simulink model "Emission_Estimator_And_Consumption_Optimizer"  (R2016b)
settings: Solver=VariableStepAuto  StartTime=0.0  StopTime=10.0  RelTol=1e-3
libraries: gtlink2017 x1
settings Model: Creator=r03schne  LastModifiedBy=r03schne

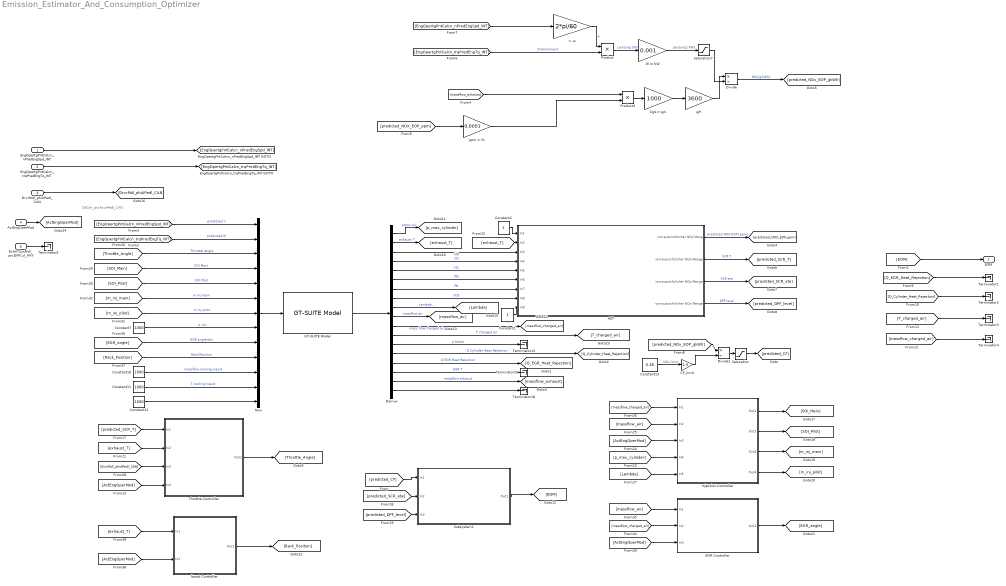
== system Emission_Estimator_And_Consumption_Optimizer ==
  note: DtCtrl_prcAccrPedl_CAN
  EngOpertgPntCalcn_nPredEngSpd_INT : Inport
  EngOpertgPntCalcn_trqPredEngTq_INT : Inport  Port=2
  DrvrMdl_phiAPedl_CAN : Inport  Port=3
  ActEngOperMod : Inport  Port=4
  ExhATSysMdl_prcDPFLvl_PHY : Inport  Port=5
  AET : Subsystem
      mask Display: image('C:\Users\r03schne\Pictures\RusspartikelFilter.jpg');
  "CF_limit " : Gain  Gain=1.5
  Constant1 : Constant
  Constant{7,10..12} (4 alike) : Constant  Value=1000
  Constant13 : Constant  Value=0.46
  Constant2 : Constant
  Demux : Demux  Outputs=18
  Divide : Product  Inputs=*/
  Divide1 : Product  Inputs=*/
  EGR Controller : Subsystem
      mask Display: image('C:\Users\r03schne\Pictures\drosselklappe_alt.png');
  GT-SUITE Model : gtlink2017/R2014b_and_higher /GT-SUITE Model  gti_fname='C:\Users\r03schne\Desktop\MAN_D26Dummymodell\D2676LF45_FRM_KF_BASIS_HARNESS-V2017.gtm'  gti_fname_warn=off  gti_dur=SIMULINK  gti_dt=0.001  gti_case=1  gti_ni=4  gti_no=18  gti_parnam='ign'  gti_parval='ign'  gti_runsimu=on  gti_coreno=1  gti_sui=console window  gti_monitors=on  gti_bits=default  gti_build=-1  gti_advanced=on  gti_halt=off  gti_initdlay=off  gti_cacomb=off  gti_ioreport=off  gti_feedthru=off  gti_add_image_to_block=Yes  gti_image_width=119  gti_image_height=139
      settings: AttributesFormatString=%<gti_fname>
  Injection Controller : Subsystem
      mask Display: image('C:\Users\r03schne\Pictures\injektor.png');
  Mux : Mux  Inputs=13
  Product : Product
  Product4 : Product
  Saturation : Saturate  UpperLimit=100  LowerLimit=0
  Saturation7 : Saturate  UpperLimit=4000  LowerLimit=1
  Subsystem1 : Subsystem
      mask Display: image('C:\Users\r03schne\Pictures\logic-1630657_960_720.png');
  Terminator{1..5,13,16,18} (8 alike) : Terminator
  Throttle Controller : Subsystem
      mask Display: image('C:\Users\r03schne\Pictures\drosselklappe_alt.png');
  W in KW : Gain  Gain=0.001
  boost Controller : Subsystem
      mask Display: image('C:\Users\r03schne\Pictures\GTX-Turbolader.jpg');
  g/h : Gain  Gain=3600
  kg/s in g/s : Gain  Gain=1000
  n -w : Gain  Gain=2*pi/60
  ppm in % : Gain  Gain=0.0001
  EOM : Outport  OutMin=0  OutMax=10  OutDataTypeStr=int8  PortDimensions="[1  1]"  SampleTime=0.01
  wires:
  GT-SUITE Model/1 -> Demux/1
  Demux/10 -> [massflow_air]  "massflow air"
  Demux/11 -> [massflow_charged_air]  "mass flow charged air"
  Mux/1 -> GT-SUITE Model/1
  Demux/12 -> [T_charged_air]  "T charged air"
  Demux/13 -> Terminator13/1  "p boost"
  Demux/14 -> [Q_Cylinder_Heat_Rejection]  "Q Cylinder Heat Rejection"
  Demux/15 -> [Q_EGR_Heat_Rejection]  "Q EGR Heat Rejection"
  Demux/16 -> Terminator16/1  "EGR T"
  Demux/17 -> [massflow_exhaust]  "massflow exhaust"
  Demux/18 -> Terminator18/1
  [Throttle_Angle] -> Mux/3  "Throttel Angle"
  [SOI_Main] -> Mux/4  "SOI Main"
  [SOI_Pilot] -> Mux/5  "SOI Pilot"
  [m_inj_main] -> Mux/6  "m inj main"
  [m_inj_pilot] -> Mux/7  "m inj pilot"
  Constant7/1 -> Mux/8  "p rail"
  [EGR_angle] -> Mux/9  "EGR angle/dm"
  [Rack_Position] -> Mux/10  "Rack-Position"
  Constant10/1 -> Mux/11  "massflow cooling_liquid"
  Constant11/1 -> Mux/12  "T cooling liquid"
  Constant12/1 -> Mux/13
  Demux/1 -> [p_max_cylinder]  "pmax cyl"
  Demux/2 -> [exhaust_T]  "exhaust T"
  Demux/3 -> AET/3(In3)  "NO"
  Demux/4 -> AET/4(In4)  "CO"
  Demux/5 -> AET/5(In5)  "HC"
  Demux/6 -> AET/6(In6)  "PM"
  Demux/7 -> AET/7(In7)  "PN"
  Demux/8 -> AET/8(In8)  "CO2"
  Demux/9 -> [Lambda]  "Lambda"
  Constant13/1 -> "CF_limit "/1  "NOx limit"
  AET/1(vorraussichtlicher NOx Menge) -> [predicted_NOX_EOP_ppm]  "predicted NOX EOP [ppm]"
  n -w/1 -> Product/1  "w"
  Product/1 -> W in KW/1  "Leistung [W]"
  [EngOpertgPntCalcn_trqPredEngTq_INT] -> Product/2  "Drehmoment"
  W in KW/1 -> Saturation7/1  "Leistung [KW]"
  ppm in %/1 -> Product4/2
  Product4/1 -> kg/s in g/s/1
  kg/s in g/s/1 -> g/h/1
  g/h/1 -> Divide/1
  Divide/1 -> [predicted_NOx_EOP_gkWh]  "NOx[g/kWh]"
  [massflow_exhaust] -> Product4/1
  Saturation7/1 -> Divide/2
  [EngOpertgPntCalcn_nPredEngSpd_INT] -> n -w/1
  [predicted_NOX_EOP_ppm] -> ppm in %/1
  [predicted_NOx_EOP_gkWh] -> Divide1/1
  "CF_limit "/1 -> Divide1/2
  Divide1/1 -> Saturation/1
  Saturation/1 -> [predicted_CF]
  AET/2(vorraussichtlicher NOx Menge1) -> [predicted_SCR_T]  "SCR T"
  AET/3(vorraussichtlicher NOx Menge2) -> [predicted_SCR_eta]  "SCR eta"
  AET/4(vorraussichtlicher NOx Menge3) -> [predicted_DPF_level]  "DPF level"
  [predicted_SCR_T] -> Throttle Controller/1(In1)
  [exhaust_T] -> Throttle Controller/2(In2)
  Throttle Controller/1(Out1) -> [Throttle_Angle]
  [exhaust_T] -> AET/2(In2)
  DrvrMdl_phiAPedl_CAN/1 -> [DrvrMdl_phiAPedl_CAN]
  [DrvrMdl_phiAPedl_CAN] -> Throttle Controller/3(In3)
  [massflow_charged_air] -> Injection Controller/1(In1)
  [massflow_air] -> Injection Controller/2(In2)
  [ActEngOperMod] -> Injection Controller/3(In3)
  [p_max_cylinder] -> Injection Controller/4(In4)
  [Lambda] -> Injection Controller/5(In5)
  Injection Controller/1(Out1) -> [SOI_Main]
  Injection Controller/2(Out2) -> [SOI_Pilot]
  Injection Controller/3(Out3) -> [m_inj_main]
  Injection Controller/4(Out4) -> [m_inj_pilot]
  [massflow_air] -> EGR Controller/1(In1)
  [massflow_charged_air] -> EGR Controller/2(In2)
  [ActEngOperMod] -> EGR Controller/3(In3)
  EGR Controller/1(Out1) -> [EGR_angle]
  [exhaust_T] -> boost Controller/1(In1)
  [ActEngOperMod] -> boost Controller/2(In2)
  boost Controller/1(Out1) -> [Rack_Position]
  Subsystem1/1(Out1) -> [EOM]
  [predicted_CF] -> Subsystem1/1(In1)
  [EOM] -> EOM/1
  EngOpertgPntCalcn_nPredEngSpd_INT/1 -> [EngOpertgPntCalcn_nPredEngSpd_INT]
  EngOpertgPntCalcn_trqPredEngTq_INT/1 -> [EngOpertgPntCalcn_trqPredEngTq_INT]
  [EngOpertgPntCalcn_nPredEngSpd_INT] -> Mux/1  "predicted n"
  [EngOpertgPntCalcn_trqPredEngTq_INT] -> Mux/2  "predicted M"
  Constant2/1 -> AET/1(In1)
  [massflow_charged_air] -> Terminator4/1
  Constant1/1 -> AET/9(In9)
  [Q_Cylinder_Heat_Rejection] -> Terminator2/1
  [Q_EGR_Heat_Rejection] -> Terminator1/1
  [T_charged_air] -> Terminator3/1
  [predicted_SCR_eta] -> Subsystem1/2(In2)
  [predicted_DPF_level] -> Subsystem1/3(In3)
  ActEngOperMod/1 -> [ActEngOperMod]
  [ActEngOperMod] -> Throttle Controller/4(In4)
  ExhATSysMdl_prcDPFLvl_PHY/1 -> Terminator5/1

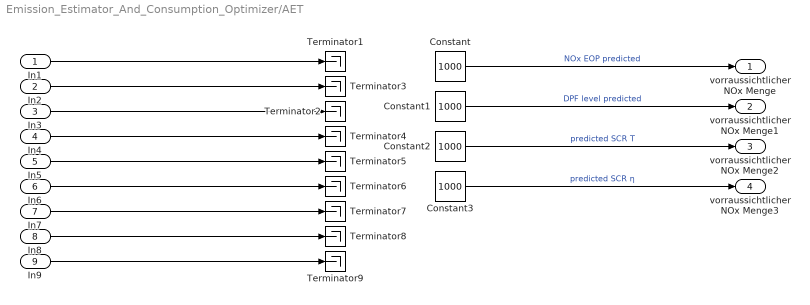
== system Emission_Estimator_And_Consumption_Optimizer/AET ==
  In1 : Inport
  In2 : Inport  Port=2
  In3 : Inport  Port=3
  In4 : Inport  Port=4
  In5 : Inport  Port=5
  In6 : Inport  Port=6
  In7 : Inport  Port=7
  In8 : Inport  Port=8
  In9 : Inport  Port=9
  Constant{,1..3} (4 alike) : Constant  Value=1000
  Terminator{1..9} (9 alike) : Terminator
  vorraussichtlicher NOx Menge : Outport
  vorraussichtlicher NOx Menge1 : Outport  Port=2
  vorraussichtlicher NOx Menge2 : Outport  Port=3
  vorraussichtlicher NOx Menge3 : Outport  Port=4
  wires:
  In3/1 -> Terminator2/1
  In2/1 -> Terminator3/1
  In4/1 -> Terminator4/1
  In5/1 -> Terminator5/1
  In6/1 -> Terminator6/1
  In7/1 -> Terminator7/1
  In8/1 -> Terminator8/1
  In9/1 -> Terminator9/1
  In1/1 -> Terminator1/1
  Constant1/1 -> vorraussichtlicher NOx Menge1/1  "DPF level predicted"
  Constant/1 -> vorraussichtlicher NOx Menge/1  "NOx EOP predicted"
  Constant2/1 -> vorraussichtlicher NOx Menge2/1  "predicted SCR T"
  Constant3/1 -> vorraussichtlicher NOx Menge3/1  "predicted SCR η"

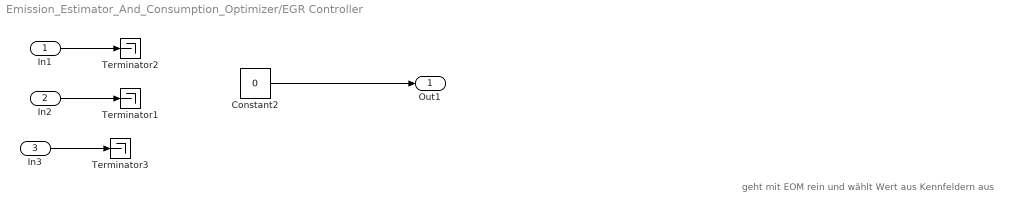
== system Emission_Estimator_And_Consumption_Optimizer/EGR Controller ==
  note: geht mit EOM rein und wählt Wert aus Kennfeldern aus
  In1 : Inport
  In2 : Inport  Port=2
  In3 : Inport  Port=3
  Constant2 : Constant  Value=0
  Terminator1 : Terminator
  Terminator2 : Terminator
  Terminator3 : Terminator
  Out1 : Outport
  wires:
  Constant2/1 -> Out1/1
  In3/1 -> Terminator3/1
  In2/1 -> Terminator1/1
  In1/1 -> Terminator2/1

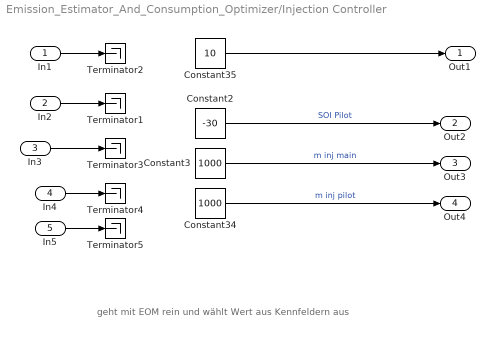
== system Emission_Estimator_And_Consumption_Optimizer/Injection Controller ==
  note: geht mit EOM rein und wählt Wert aus Kennfeldern aus
  In1 : Inport
  In2 : Inport  Port=2
  In3 : Inport  Port=3
  In4 : Inport  Port=4
  In5 : Inport  Port=5
  Constant2 : Constant  Value=-30
  Constant3 : Constant  Value=1000
  Constant34 : Constant  Value=1000
  Constant35 : Constant  Value=10
  Terminator{1..5} (5 alike) : Terminator
  Out1 : Outport
  Out2 : Outport  Port=2
  Out3 : Outport  Port=3
  Out4 : Outport  Port=4
  wires:
  Constant35/1 -> Out1/1
  Constant3/1 -> Out3/1  "m inj main"
  Constant34/1 -> Out4/1  "m inj pilot"
  Constant2/1 -> Out2/1  "SOI Pilot"
  In5/1 -> Terminator5/1
  In3/1 -> Terminator3/1
  In4/1 -> Terminator4/1
  In1/1 -> Terminator2/1
  In2/1 -> Terminator1/1

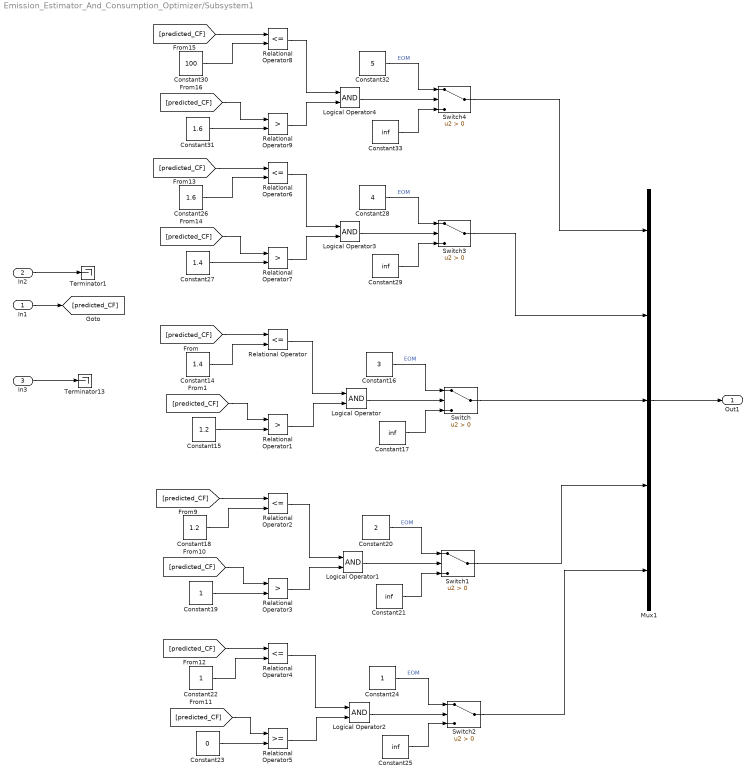
== system Emission_Estimator_And_Consumption_Optimizer/Subsystem1 ==
  In1 : Inport
  In2 : Inport  Port=2
  In3 : Inport  Port=3
  Constant14 : Constant  Value=1.4
  Constant15 : Constant  Value=1.2
  Constant16 : Constant  Value=3
  Constant{17,21,25,29,33} (5 alike) : Constant  Value=inf
  Constant18 : Constant  Value=1.2
  Constant19 : Constant
  Constant20 : Constant  Value=2
  Constant22 : Constant
  Constant23 : Constant  Value=0
  Constant24 : Constant
  Constant26 : Constant  Value=1.6
  Constant27 : Constant  Value=1.4
  Constant28 : Constant  Value=4
  Constant30 : Constant  Value=100
  Constant31 : Constant  Value=1.6
  Constant32 : Constant  Value=5
  Logical Operator{,1..4} (5 alike) : Logic  AllPortsSameDT=off  OutDataTypeStr=boolean
  Mux1 : Mux  Inputs=5
  Relational Operator{,2,4,6,8} (5 alike) : RelationalOperator  Operator=<=  OutDataTypeStr=boolean  RndMeth=Simplest
  Relational Operator{1,3,7,9} (4 alike) : RelationalOperator  Operator=>  OutDataTypeStr=boolean  RndMeth=Simplest
  Relational Operator5 : RelationalOperator  OutDataTypeStr=boolean  RndMeth=Simplest
  Switch{,1..4} (5 alike) : Switch  Criteria=u2 > Threshold
  Terminator1 : Terminator
  Terminator13 : Terminator
  Out1 : Outport
  wires:
  [predicted_CF] -> Relational Operator4/1
  Relational Operator7/1 -> Logical Operator3/2
  Switch/1 -> Mux1/3
  Relational Operator9/1 -> Logical Operator4/2
  [predicted_CF] -> Relational Operator8/1
  Relational Operator6/1 -> Logical Operator3/1
  Constant23/1 -> Relational Operator5/2
  Switch3/1 -> Mux1/2
  Constant27/1 -> Relational Operator7/2
  [predicted_CF] -> Relational Operator9/1
  Constant31/1 -> Relational Operator9/2
  Logical Operator2/1 -> Switch2/2
  Constant33/1 -> Switch4/3
  Switch2/1 -> Mux1/5
  [predicted_CF] -> Relational Operator6/1
  Constant21/1 -> Switch1/3
  Constant30/1 -> Relational Operator8/2
  Logical Operator4/1 -> Switch4/2
  Constant24/1 -> Switch2/1  "EOM"
  Constant25/1 -> Switch2/3
  Constant28/1 -> Switch3/1  "EOM"
  Relational Operator5/1 -> Logical Operator2/2
  Constant32/1 -> Switch4/1  "EOM"
  [predicted_CF] -> Relational Operator7/1
  Constant29/1 -> Switch3/3
  Relational Operator4/1 -> Logical Operator2/1
  Constant26/1 -> Relational Operator6/2
  Logical Operator3/1 -> Switch3/2
  Switch4/1 -> Mux1/1
  Switch1/1 -> Mux1/4
  Mux1/1 -> Out1/1
  [predicted_CF] -> Relational Operator5/1
  Relational Operator8/1 -> Logical Operator4/1
  Constant22/1 -> Relational Operator4/2
  Constant16/1 -> Switch/1  "EOM"
  [predicted_CF] -> Relational Operator2/1
  Relational Operator1/1 -> Logical Operator/2
  Relational Operator2/1 -> Logical Operator1/1
  Constant14/1 -> Relational Operator/2
  Constant18/1 -> Relational Operator2/2
  Constant19/1 -> Relational Operator3/2
  Constant20/1 -> Switch1/1  "EOM"
  Constant15/1 -> Relational Operator1/2
  [predicted_CF] -> Relational Operator1/1
  Constant17/1 -> Switch/3
  Relational Operator3/1 -> Logical Operator1/2
  Logical Operator/1 -> Switch/2
  Logical Operator1/1 -> Switch1/2
  [predicted_CF] -> Relational Operator/1
  [predicted_CF] -> Relational Operator3/1
  Relational Operator/1 -> Logical Operator/1
  In1/1 -> [predicted_CF]
  In2/1 -> Terminator1/1
  In3/1 -> Terminator13/1

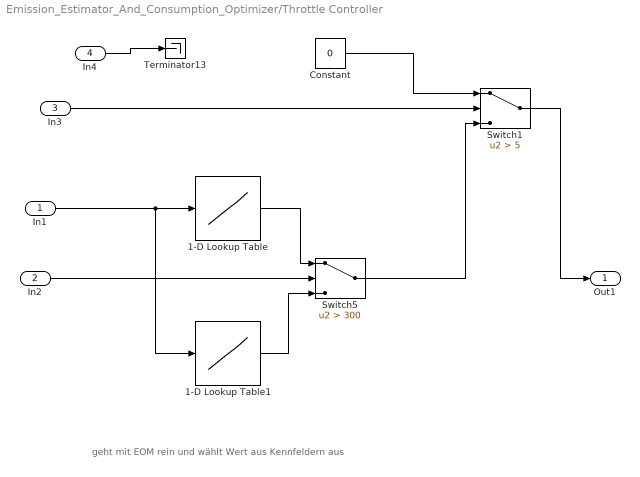
== system Emission_Estimator_And_Consumption_Optimizer/Throttle Controller ==
  note: geht mit EOM rein und wählt Wert aus Kennfeldern aus
  In1 : Inport
  In2 : Inport  Port=2
  In3 : Inport  Port=3
  In4 : Inport  Port=4
  1-D Lookup Table : Lookup_n-D  NumberOfTableDimensions=1  BreakpointsForDimension1=[0 50 100 150 200 250]  Table=[60 40 20 10 0 0]  InternalRulePriority=Speed  RndMeth=Simplest  InputSameDT=on
  1-D Lookup Table1 : Lookup_n-D  NumberOfTableDimensions=1  BreakpointsForDimension1=[0 50 100 150 200 250]  Table=[70 50 30 20 0 0]  InternalRulePriority=Speed  RndMeth=Simplest  InputSameDT=on
  Constant : Constant  Value=0
  Switch1 : Switch  Criteria=u2 > Threshold  Threshold=5
  Switch5 : Switch  Criteria=u2 > Threshold  Threshold=300
  Terminator13 : Terminator
  Out1 : Outport
  wires:
  In2/1 -> Switch5/2
  1-D Lookup Table1/1 -> Switch5/3
  1-D Lookup Table/1 -> Switch5/1
  In1/1 -> 1-D Lookup Table1/1, 1-D Lookup Table/1
  Switch5/1 -> Switch1/3
  In3/1 -> Switch1/2
  Switch1/1 -> Out1/1
  Constant/1 -> Switch1/1
  In4/1 -> Terminator13/1

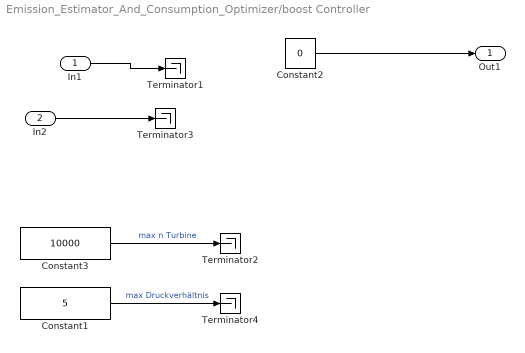
== system Emission_Estimator_And_Consumption_Optimizer/boost Controller ==
  In1 : Inport
  In2 : Inport  Port=2
  Constant1 : Constant  Value=5
  Constant2 : Constant  Value=0
  Constant3 : Constant  Value=10000
  Terminator{1..4} (4 alike) : Terminator
  Out1 : Outport
  wires:
  In2/1 -> Terminator3/1
  Constant2/1 -> Out1/1
  In1/1 -> Terminator1/1
  Constant3/1 -> Terminator2/1  "max n Turbine"
  Constant1/1 -> Terminator4/1  "max Druckverhältnis"
